simulink model "LoFT_Example3"  (R2024b)
settings: Solver=ode4  StartTime=0.0  StopTime=300  FixedStep=simu.dt  RelTol=1e-3
undefined symbols (not defined in the file): body, circtime, Communication, D1, Delta, irkb, line, LoFT, p0, Pn, s, simu, trip_time, Turbwind, waves, wind
libraries: simulink x350, spsThreePhaseVIMeasurementLib x41, spsThreePhasePISectionLineLib x34, spsThreePhaseParallelRLCLoadLib x21, spsThreePhaseTransformerTwoWindingsLib x14, spsLoadFlowBusLib x10, spsThreePhaseDynamicLoadLib x9, spsSynchronousMachinepuStandardLib x7, spsExcitationSystemLib x7, spsSteamTurbineandGovernorLib x7, spsGenericPowerSystemStabilizerLib x7, spsMultiBandPowerSystemStabilizerLib x7
(part 22 of 49)

== system LoFT_Example3/FOWT System/Subsystem5/FOWT5/Aerodynamics and Local Control Systems ==
  WindSpeed : Inport
  "Measureed " : Inport  Port=2
  Nacelle Speed : Inport  Port=3
  Power : Inport  Port=4
  Blade Pitch : Inport  Port=5
  Switch : Inport  Port=6
  Constant1 : Constant  Value=90*pi/180
  Demux : Demux  Outputs=2
  Divide3 : Product  Inputs=*/
  Hull Aerodynamic : Subsystem
  Local Control Systems : Subsystem
  Mux : Mux
  Mux1 : Mux
  Product : Product
  Rate Limiter : RateLimiter  RisingSlewLimit=Controller.torqueMaxRate  FallingSlewLimit=-Controller.torqueMaxRate  SampleTimeMode=inherited
  Rotor/drivetrain dynamics : Subsystem
  Saturation Dynamic : simulink/Discontinuities/Saturation Dynamic  OutMin=[]  OutMax=[]  OutDataTypeStr=Inherit: Same as second input  OutDataType=fixdt(1, 16)  OutScaling=2^-10  DoSatur=off
  Saturation2 : Saturate  UpperLimit=Controller.torqueMax  LowerLimit=0
  Switch1 : Switch  Criteria=u2 > Threshold  SaturateOnIntegerOverflow=off  InputSameDT=off
  Transfer Fcn : TransferFcn  Denominator=[0.2 1]
  smooth1 : Subsystem
  wind speed estimator : Subsystem
  Nacelle : Outport
  drivetrain : Outport  Port=2
  F_aero : Outport  Port=3
  wires:
  Transfer Fcn/1 -> [BldPitch]
  Mux1/1 -> drivetrain/1
  Mux/1 -> Nacelle/1
  Local Control Systems/2(BldPitch) -> Saturation Dynamic/2
  Saturation Dynamic/1 -> Transfer Fcn/1
  Switch/1 -> Demux/1
  [RotSpeed] -> Divide3/2
  Rate Limiter/1 -> Saturation2/1
  Switch1/1 -> Rate Limiter/1
  Local Control Systems/1(GenTorq) -> Switch1/3
  Divide3/1 -> Switch1/1
  Nacelle Speed/1 -> Local Control Systems/3(Nacelle Speed)
  [RotSpeed] -> Local Control Systems/2(RotSpeed)
  Power/1 -> smooth1/1(In1)
  Blade Pitch/1 -> Saturation Dynamic/3
  Saturation2/1 -> [GenTorq]
  smooth1/1(Out1) -> Divide3/1
  WindSpeed/1 -> [EffectiveWS]
  [EffectiveWS] -> Hull Aerodynamic/1(In1)
  [RotSpeed] -> Hull Aerodynamic/2(In2)
  [BldPitch] -> Hull Aerodynamic/3(In4)
  Hull Aerodynamic/1(Out1) -> F_aero/1
  [RotSpeed] -> Rotor/drivetrain dynamics/1(In1)
  [EffectiveWS] -> Rotor/drivetrain dynamics/2(In2)
  [BldPitch] -> Rotor/drivetrain dynamics/3(In3)
  [EffectiveWS] -> Rotor/drivetrain dynamics/4(In4)
  [GenTorq] -> Rotor/drivetrain dynamics/5(In5)
  Rotor/drivetrain dynamics/1(Out1) -> [RotSpeed]
  [EffectiveWS] -> Mux/1
  [MeasuredWS] -> Local Control Systems/1(WindSpeed)
  "Measureed "/1 -> [MeasuredWS]
  [MeasuredWS] -> wind speed estimator/1(In1)
  wind speed estimator/1(Out1) -> Mux/2
  [BldPitch] -> Mux/4
  Hull Aerodynamic/2(Rotor thrust) -> [RotorThrust]
  [RotorThrust] -> Mux/3
  Demux/1 -> Switch1/2
  [RotSpeed] -> Mux1/1, Product/1
  [GenTorq] -> Mux1/2, Product/2
  Product/1 -> Mux1/3
  Rotor/drivetrain dynamics/2(Out2) -> [RotTorq]
  [RotTorq] -> Mux1/4
  Constant1/1 -> Saturation Dynamic/1

== system LoFT_Example3/FOWT System/Subsystem5/FOWT5/Hydrodynamics ==
  Acceleration : Inport
  Speed : Inport  Port=2
  Position : Inport  Port=3
  Wave : Inport  Port=4
  Add : Sum  Inputs=--+
  excitation force : Subsystem
  radiation force : Subsystem
  "viscous force " : Subsystem
  Out1 : Outport
  wires:
  Wave/1 -> excitation force/2(Wave)
  Add/1 -> Out1/1
  excitation force/1(Fext) -> Add/3
  "viscous force "/1(F_vis) -> Add/2
  radiation force/1(F_rad) -> Add/1
  Position/1 -> excitation force/1(position)
  Acceleration/1 -> radiation force/1(velocity)
  Speed/1 -> "viscous force "/1(In1), radiation force/2(In2)

== system LoFT_Example3/FOWT System/Subsystem5/FOWT5/Hydrostatics ==
  position : Inport
  Add : Sum
  Add2 : Sum  Inputs=+--
  Assignment : Assignment  DiagnosticForDimensions=Warning  IndexOptions=Index vector (dialog)  Indices=2  OutputSizes=1
  Constant : Constant  Value=Property.masstot-9.7e6
  Constant1 : Constant  Value=Property.volume
  Constant2 : Constant  Value=[0 0 0]
  Constant3 : Constant  Value=4*445087
  Product : Product  Multiplication=Matrix(*)
  "Surge,heave,pitch, Hydro stiffness (3×3)" : Constant  Value=Hydro.hydrostatic
  rho * g : Gain  Gain=1025*9.81
  rho * g1 : Gain  Gain=9.81
  Out1 : Outport
  wires:
  Add2/1 -> Assignment/2
  Add/1 -> Out1/1
  Assignment/1 -> Add/1
  Constant2/1 -> Assignment/1
  rho * g/1 -> Add2/2
  rho * g1/1 -> Add2/1
  Constant/1 -> rho * g1/1
  Product/1 -> Add/2
  Constant1/1 -> rho * g/1
  position/1 -> Product/2
  "Surge,heave,pitch, Hydro stiffness (3×3)"/1 -> Product/1
  Constant3/1 -> Add2/3

== system LoFT_Example3/FOWT System/Subsystem5/FOWT5/Measurements ==
  Nacelle : Inport
  drivetrain : Inport  Port=2
  platform : Inport  Port=3
  Bus Creator : BusCreator  Inputs=17
  Demux : Demux  Outputs=9
  Demux1 : Demux
  Demux2 : Demux
  Out1 : Outport
  wires:
  drivetrain/1 -> Demux2/1
  Demux2/4 -> Bus Creator/8  "RotTorq"
  Demux2/3 -> Bus Creator/7  "GenPwr"
  Demux2/2 -> Bus Creator/6  "GenTorq"
  Demux2/1 -> Bus Creator/5  "RotSpeed"
  Demux/1 -> Bus Creator/9  "PtfmSurge"
  Demux/2 -> Bus Creator/10  "PtfmHeave"
  Demux/3 -> Bus Creator/11  "PtfmPitch"
  Demux/4 -> Bus Creator/12  "PtfmTVxi"
  Demux/5 -> Bus Creator/13  "PtfmTVzi"
  Demux/6 -> Bus Creator/14  "PtfmRVyi"
  Demux/7 -> Bus Creator/15  "PtfmTAxi"
  Demux/8 -> Bus Creator/16  "PtfmTAzi"
  Demux/9 -> Bus Creator/17  "PtfmRAyi"
  Demux1/1 -> Bus Creator/1  "WindVelX"
  Demux1/2 -> Bus Creator/2  "WindEst"
  Demux1/3 -> Bus Creator/3  "RotThrust"
  Demux1/4 -> Bus Creator/4  "BldPitch"
  Bus Creator/1 -> Out1/1
  Nacelle/1 -> Demux1/1
  platform/1 -> Demux/1

== system LoFT_Example3/FOWT System/Subsystem5/FOWT5/Moorings ==
  position : Inport
  2-D Lookup Table : Lookup_n-D  NumberOfTableDimensions=3  BreakpointsForDimension1=Mooring.X  BreakpointsForDimension2=Mooring.Z  BreakpointsForDimension3=Mooring.RY  Table=Mooring.FX  InternalRulePriority=Speed  RndMeth=Simplest
      settings: InputPortMap=u0,u1,u2
  2-D Lookup Table3 : Lookup_n-D  NumberOfTableDimensions=3  BreakpointsForDimension1=LoFT.Mooring.X  BreakpointsForDimension2=LoFT.Mooring.Z  BreakpointsForDimension3=LoFT.Mooring.RY  Table=LoFT.Mooring.FZ  InternalRulePriority=Speed  RndMeth=Simplest
      settings: InputPortMap=u0,u1,u2
  2-D Lookup Table4 : Lookup_n-D  NumberOfTableDimensions=3  BreakpointsForDimension1=LoFT.Mooring.X  BreakpointsForDimension2=LoFT.Mooring.Z  BreakpointsForDimension3=LoFT.Mooring.RY  Table=LoFT.Mooring.MY  InternalRulePriority=Speed  RndMeth=Simplest
      settings: InputPortMap=u0,u1,u2
  Demux : Demux  Outputs=3
  Demux1 : Demux  Outputs=3
  Demux2 : Demux  Outputs=3
  Vector Concatenate1 : Concatenate  NumInputs=3
  Out1 : Outport
  wires:
  Vector Concatenate1/1 -> Out1/1
  Demux2/2 -> 2-D Lookup Table4/2
  Demux2/1 -> 2-D Lookup Table4/1
  2-D Lookup Table4/1 -> Vector Concatenate1/3
  2-D Lookup Table3/1 -> Vector Concatenate1/2
  Demux1/3 -> 2-D Lookup Table3/3
  Demux/2 -> 2-D Lookup Table/2
  Demux1/1 -> 2-D Lookup Table3/1
  Demux2/3 -> 2-D Lookup Table4/3
  Demux/1 -> 2-D Lookup Table/1
  position/1 -> Demux/1, Demux1/1, Demux2/1
  2-D Lookup Table/1 -> Vector Concatenate1/1
  Demux1/2 -> 2-D Lookup Table3/2
  Demux/3 -> 2-D Lookup Table/3

== system LoFT_Example3/FOWT System/Subsystem5/FOWT5/Subsystem1 ==
  In1 : Inport
  In2 : Inport  Port=2
  In3 : Inport  Port=3
  In4 : Inport  Port=4
  In5 : Inport  Port=5
  In6 : Inport  Port=6
  Demux : Demux  Outputs=2
  Demux1 : Demux  Outputs=2
  Demux2 : Demux  Outputs=2
  Mux : Mux  Inputs=9
  Vector Concatenate : Concatenate
  Vector Concatenate1 : Concatenate
  Vector Concatenate2 : Concatenate
  Out4 : Outport
  Out1 : Outport  Port=2
  Out2 : Outport  Port=3
  Out3 : Outport  Port=4
  wires:
  Demux2/2 -> Mux/8
  Demux2/1 -> Mux/7
  Demux1/2 -> Mux/5
  Demux1/1 -> Mux/4
  Demux/2 -> Mux/2
  Demux/1 -> Mux/1
  Mux/1 -> Out4/1
  In6/1 -> Vector Concatenate2/1, Demux2/1
  In2/1 -> Vector Concatenate1/2, Mux/6
  In5/1 -> Vector Concatenate1/1, Demux1/1
  Vector Concatenate/1 -> Out1/1
  Vector Concatenate1/1 -> Out2/1
  Vector Concatenate2/1 -> Out3/1
  In4/1 -> Vector Concatenate/1, Demux/1
  In1/1 -> Vector Concatenate/2, Mux/3
  In3/1 -> Vector Concatenate2/2, Mux/9

== system LoFT_Example3/FOWT System/Subsystem5/FOWT5/wind speed(m//s) ==
  Inflow : Inport
  In2 : Inport  Port=2
  Add : Sum
  Demux : Demux  Outputs=3
  Product : Product
  Trigonometric Function : Trigonometry  Operator=cos
  add : Sum  Inputs=+-
  add1 : Sum  Inputs=+-
  hub height : Gain  Gain=145
  smooth1 : Subsystem  Commented=on
  Effective : Outport
  Measured : Outport  Port=2
  FB : Outport  Port=3
  wires:
  In2/1 -> Demux/1
  hub height/1 -> Product/1
  Trigonometric Function/1 -> Product/2
  Demux/1 -> Add/1
  Demux/3 -> hub height/1, Trigonometric Function/1
  add/1 -> Effective/1
  add1/1 -> Measured/1
  Product/1 -> Add/2
  Add/1 -> [HubVelocity]
  [HubVelocity] -> add1/2
  [HubVelocity] -> add/2
  [HubVelocity] -> FB/1
  Inflow/1 -> add1/1, add/1

== system LoFT_Example3/FOWT System/Subsystem5/FOWT6/Aerodynamics and Local Control Systems ==
  WindSpeed : Inport
  "Measureed " : Inport  Port=2
  Nacelle Speed : Inport  Port=3
  Power : Inport  Port=4
  Blade Pitch : Inport  Port=5
  Switch : Inport  Port=6
  Constant1 : Constant  Value=90*pi/180
  Demux : Demux  Outputs=2
  Divide3 : Product  Inputs=*/
  Hull Aerodynamic : Subsystem
  Local Control Systems : Subsystem
  Mux : Mux
  Mux1 : Mux
  Product : Product
  Rate Limiter : RateLimiter  RisingSlewLimit=Controller.torqueMaxRate  FallingSlewLimit=-Controller.torqueMaxRate  SampleTimeMode=inherited
  Rotor/drivetrain dynamics : Subsystem
  Saturation Dynamic : simulink/Discontinuities/Saturation Dynamic  OutMin=[]  OutMax=[]  OutDataTypeStr=Inherit: Same as second input  OutDataType=fixdt(1, 16)  OutScaling=2^-10  DoSatur=off
  Saturation2 : Saturate  UpperLimit=Controller.torqueMax  LowerLimit=0
  Switch1 : Switch  Criteria=u2 > Threshold  SaturateOnIntegerOverflow=off  InputSameDT=off
  Transfer Fcn : TransferFcn  Denominator=[0.2 1]
  smooth1 : Subsystem
  wind speed estimator : Subsystem
  Nacelle : Outport
  drivetrain : Outport  Port=2
  F_aero : Outport  Port=3
  wires:
  Constant1/1 -> Saturation Dynamic/1
  [RotTorq] -> Mux1/4
  Rotor/drivetrain dynamics/2(Out2) -> [RotTorq]
  Product/1 -> Mux1/3
  [GenTorq] -> Product/2, Mux1/2
  [RotSpeed] -> Product/1, Mux1/1
  Demux/1 -> Switch1/2
  [RotorThrust] -> Mux/3
  Hull Aerodynamic/2(Rotor thrust) -> [RotorThrust]
  [BldPitch] -> Mux/4
  wind speed estimator/1(Out1) -> Mux/2
  [MeasuredWS] -> wind speed estimator/1(In1)
  "Measureed "/1 -> [MeasuredWS]
  [MeasuredWS] -> Local Control Systems/1(WindSpeed)
  [EffectiveWS] -> Mux/1
  Rotor/drivetrain dynamics/1(Out1) -> [RotSpeed]
  [GenTorq] -> Rotor/drivetrain dynamics/5(In5)
  [EffectiveWS] -> Rotor/drivetrain dynamics/4(In4)
  [BldPitch] -> Rotor/drivetrain dynamics/3(In3)
  [EffectiveWS] -> Rotor/drivetrain dynamics/2(In2)
  [RotSpeed] -> Rotor/drivetrain dynamics/1(In1)
  Hull Aerodynamic/1(Out1) -> F_aero/1
  [BldPitch] -> Hull Aerodynamic/3(In4)
  [RotSpeed] -> Hull Aerodynamic/2(In2)
  [EffectiveWS] -> Hull Aerodynamic/1(In1)
  WindSpeed/1 -> [EffectiveWS]
  smooth1/1(Out1) -> Divide3/1
  Saturation2/1 -> [GenTorq]
  Blade Pitch/1 -> Saturation Dynamic/3
  Power/1 -> smooth1/1(In1)
  [RotSpeed] -> Local Control Systems/2(RotSpeed)
  Nacelle Speed/1 -> Local Control Systems/3(Nacelle Speed)
  Divide3/1 -> Switch1/1
  Local Control Systems/1(GenTorq) -> Switch1/3
  Switch1/1 -> Rate Limiter/1
  Rate Limiter/1 -> Saturation2/1
  [RotSpeed] -> Divide3/2
  Switch/1 -> Demux/1
  Saturation Dynamic/1 -> Transfer Fcn/1
  Local Control Systems/2(BldPitch) -> Saturation Dynamic/2
  Mux/1 -> Nacelle/1
  Mux1/1 -> drivetrain/1
  Transfer Fcn/1 -> [BldPitch]

== system LoFT_Example3/FOWT System/Subsystem5/FOWT6/Hydrodynamics ==
  Acceleration : Inport
  Speed : Inport  Port=2
  Position : Inport  Port=3
  Wave : Inport  Port=4
  Add : Sum  Inputs=--+
  excitation force : Subsystem
  radiation force : Subsystem
  "viscous force " : Subsystem
  Out1 : Outport
  wires:
  Speed/1 -> radiation force/2(In2), "viscous force "/1(In1)
  Acceleration/1 -> radiation force/1(velocity)
  Position/1 -> excitation force/1(position)
  radiation force/1(F_rad) -> Add/1
  "viscous force "/1(F_vis) -> Add/2
  excitation force/1(Fext) -> Add/3
  Add/1 -> Out1/1
  Wave/1 -> excitation force/2(Wave)

== system LoFT_Example3/FOWT System/Subsystem5/FOWT6/Hydrostatics ==
  position : Inport
  Add : Sum
  Add2 : Sum  Inputs=+--
  Assignment : Assignment  DiagnosticForDimensions=Warning  IndexOptions=Index vector (dialog)  Indices=2  OutputSizes=1
  Constant : Constant  Value=Property.masstot-9.7e6
  Constant1 : Constant  Value=Property.volume
  Constant2 : Constant  Value=[0 0 0]
  Constant3 : Constant  Value=4*445087
  Product : Product  Multiplication=Matrix(*)
  "Surge,heave,pitch, Hydro stiffness (3×3)" : Constant  Value=Hydro.hydrostatic
  rho * g : Gain  Gain=1025*9.81
  rho * g1 : Gain  Gain=9.81
  Out1 : Outport
  wires:
  Constant3/1 -> Add2/3
  "Surge,heave,pitch, Hydro stiffness (3×3)"/1 -> Product/1
  position/1 -> Product/2
  Constant1/1 -> rho * g/1
  Product/1 -> Add/2
  Constant/1 -> rho * g1/1
  rho * g1/1 -> Add2/1
  rho * g/1 -> Add2/2
  Constant2/1 -> Assignment/1
  Assignment/1 -> Add/1
  Add/1 -> Out1/1
  Add2/1 -> Assignment/2

== system LoFT_Example3/FOWT System/Subsystem5/FOWT6/Measurements ==
  Nacelle : Inport
  drivetrain : Inport  Port=2
  platform : Inport  Port=3
  Bus Creator : BusCreator  Inputs=17
  Demux : Demux  Outputs=9
  Demux1 : Demux
  Demux2 : Demux
  Out1 : Outport
  wires:
  platform/1 -> Demux/1
  Nacelle/1 -> Demux1/1
  Bus Creator/1 -> Out1/1
  Demux1/4 -> Bus Creator/4  "BldPitch"
  Demux1/3 -> Bus Creator/3  "RotThrust"
  Demux1/2 -> Bus Creator/2  "WindEst"
  Demux1/1 -> Bus Creator/1  "WindVelX"
  Demux/9 -> Bus Creator/17  "PtfmRAyi"
  Demux/8 -> Bus Creator/16  "PtfmTAzi"
  Demux/7 -> Bus Creator/15  "PtfmTAxi"
  Demux/6 -> Bus Creator/14  "PtfmRVyi"
  Demux/5 -> Bus Creator/13  "PtfmTVzi"
  Demux/4 -> Bus Creator/12  "PtfmTVxi"
  Demux/3 -> Bus Creator/11  "PtfmPitch"
  Demux/2 -> Bus Creator/10  "PtfmHeave"
  Demux/1 -> Bus Creator/9  "PtfmSurge"
  Demux2/1 -> Bus Creator/5  "RotSpeed"
  Demux2/2 -> Bus Creator/6  "GenTorq"
  Demux2/3 -> Bus Creator/7  "GenPwr"
  Demux2/4 -> Bus Creator/8  "RotTorq"
  drivetrain/1 -> Demux2/1

== system LoFT_Example3/FOWT System/Subsystem5/FOWT6/Moorings ==
  position : Inport
  2-D Lookup Table : Lookup_n-D  NumberOfTableDimensions=3  BreakpointsForDimension1=Mooring.X  BreakpointsForDimension2=Mooring.Z  BreakpointsForDimension3=Mooring.RY  Table=Mooring.FX  InternalRulePriority=Speed  RndMeth=Simplest
      settings: InputPortMap=u0,u1,u2
  2-D Lookup Table3 : Lookup_n-D  NumberOfTableDimensions=3  BreakpointsForDimension1=LoFT.Mooring.X  BreakpointsForDimension2=LoFT.Mooring.Z  BreakpointsForDimension3=LoFT.Mooring.RY  Table=LoFT.Mooring.FZ  InternalRulePriority=Speed  RndMeth=Simplest
      settings: InputPortMap=u0,u1,u2
  2-D Lookup Table4 : Lookup_n-D  NumberOfTableDimensions=3  BreakpointsForDimension1=LoFT.Mooring.X  BreakpointsForDimension2=LoFT.Mooring.Z  BreakpointsForDimension3=LoFT.Mooring.RY  Table=LoFT.Mooring.MY  InternalRulePriority=Speed  RndMeth=Simplest
      settings: InputPortMap=u0,u1,u2
  Demux : Demux  Outputs=3
  Demux1 : Demux  Outputs=3
  Demux2 : Demux  Outputs=3
  Vector Concatenate1 : Concatenate  NumInputs=3
  Out1 : Outport
  wires:
  Demux/3 -> 2-D Lookup Table/3
  Demux1/2 -> 2-D Lookup Table3/2
  2-D Lookup Table/1 -> Vector Concatenate1/1
  position/1 -> Demux2/1, Demux1/1, Demux/1
  Demux/1 -> 2-D Lookup Table/1
  Demux2/3 -> 2-D Lookup Table4/3
  Demux1/1 -> 2-D Lookup Table3/1
  Demux/2 -> 2-D Lookup Table/2
  Demux1/3 -> 2-D Lookup Table3/3
  2-D Lookup Table3/1 -> Vector Concatenate1/2
  2-D Lookup Table4/1 -> Vector Concatenate1/3
  Demux2/1 -> 2-D Lookup Table4/1
  Demux2/2 -> 2-D Lookup Table4/2
  Vector Concatenate1/1 -> Out1/1

== system LoFT_Example3/FOWT System/Subsystem5/FOWT6/Subsystem1 ==
  In1 : Inport
  In2 : Inport  Port=2
  In3 : Inport  Port=3
  In4 : Inport  Port=4
  In5 : Inport  Port=5
  In6 : Inport  Port=6
  Demux : Demux  Outputs=2
  Demux1 : Demux  Outputs=2
  Demux2 : Demux  Outputs=2
  Mux : Mux  Inputs=9
  Vector Concatenate : Concatenate
  Vector Concatenate1 : Concatenate
  Vector Concatenate2 : Concatenate
  Out4 : Outport
  Out1 : Outport  Port=2
  Out2 : Outport  Port=3
  Out3 : Outport  Port=4
  wires:
  In3/1 -> Mux/9, Vector Concatenate2/2
  In1/1 -> Mux/3, Vector Concatenate/2
  In4/1 -> Demux/1, Vector Concatenate/1
  Vector Concatenate2/1 -> Out3/1
  Vector Concatenate1/1 -> Out2/1
  Vector Concatenate/1 -> Out1/1
  In5/1 -> Demux1/1, Vector Concatenate1/1
  In2/1 -> Mux/6, Vector Concatenate1/2
  In6/1 -> Demux2/1, Vector Concatenate2/1
  Mux/1 -> Out4/1
  Demux/1 -> Mux/1
  Demux/2 -> Mux/2
  Demux1/1 -> Mux/4
  Demux1/2 -> Mux/5
  Demux2/1 -> Mux/7
  Demux2/2 -> Mux/8

== system LoFT_Example3/FOWT System/Subsystem5/FOWT6/wind speed(m//s) ==
  Inflow : Inport
  In2 : Inport  Port=2
  Add : Sum
  Demux : Demux  Outputs=3
  Product : Product
  Trigonometric Function : Trigonometry  Operator=cos
  add : Sum  Inputs=+-
  add1 : Sum  Inputs=+-
  hub height : Gain  Gain=145
  smooth1 : Subsystem  Commented=on
  Effective : Outport
  Measured : Outport  Port=2
  FB : Outport  Port=3
  wires:
  Inflow/1 -> add/1, add1/1
  [HubVelocity] -> FB/1
  [HubVelocity] -> add/2
  [HubVelocity] -> add1/2
  Add/1 -> [HubVelocity]
  Product/1 -> Add/2
  add1/1 -> Measured/1
  add/1 -> Effective/1
  Demux/3 -> Trigonometric Function/1, hub height/1
  Demux/1 -> Add/1
  Trigonometric Function/1 -> Product/2
  hub height/1 -> Product/1
  In2/1 -> Demux/1

== system LoFT_Example3/FOWT System/Subsystem5/FOWT7/Aerodynamics and Local Control Systems ==
  WindSpeed : Inport
  "Measureed " : Inport  Port=2
  Nacelle Speed : Inport  Port=3
  Power : Inport  Port=4
  Blade Pitch : Inport  Port=5
  Switch : Inport  Port=6
  Constant1 : Constant  Value=90*pi/180
  Demux : Demux  Outputs=2
  Divide3 : Product  Inputs=*/
  Hull Aerodynamic : Subsystem
  Local Control Systems : Subsystem
  Mux : Mux
  Mux1 : Mux
  Product : Product
  Rate Limiter : RateLimiter  RisingSlewLimit=Controller.torqueMaxRate  FallingSlewLimit=-Controller.torqueMaxRate  SampleTimeMode=inherited
  Rotor/drivetrain dynamics : Subsystem
  Saturation Dynamic : simulink/Discontinuities/Saturation Dynamic  OutMin=[]  OutMax=[]  OutDataTypeStr=Inherit: Same as second input  OutDataType=fixdt(1, 16)  OutScaling=2^-10  DoSatur=off
  Saturation2 : Saturate  UpperLimit=Controller.torqueMax  LowerLimit=0
  Switch1 : Switch  Criteria=u2 > Threshold  SaturateOnIntegerOverflow=off  InputSameDT=off
  Transfer Fcn : TransferFcn  Denominator=[0.2 1]
  smooth1 : Subsystem
  wind speed estimator : Subsystem
  Nacelle : Outport
  drivetrain : Outport  Port=2
  F_aero : Outport  Port=3
  wires:
  Transfer Fcn/1 -> [BldPitch]
  Mux1/1 -> drivetrain/1
  Mux/1 -> Nacelle/1
  Local Control Systems/2(BldPitch) -> Saturation Dynamic/2
  Saturation Dynamic/1 -> Transfer Fcn/1
  Switch/1 -> Demux/1
  [RotSpeed] -> Divide3/2
  Rate Limiter/1 -> Saturation2/1
  Switch1/1 -> Rate Limiter/1
  Local Control Systems/1(GenTorq) -> Switch1/3
  Divide3/1 -> Switch1/1
  Nacelle Speed/1 -> Local Control Systems/3(Nacelle Speed)
  [RotSpeed] -> Local Control Systems/2(RotSpeed)
  Power/1 -> smooth1/1(In1)
  Blade Pitch/1 -> Saturation Dynamic/3
  Saturation2/1 -> [GenTorq]
  smooth1/1(Out1) -> Divide3/1
  WindSpeed/1 -> [EffectiveWS]
  [EffectiveWS] -> Hull Aerodynamic/1(In1)
  [RotSpeed] -> Hull Aerodynamic/2(In2)
  [BldPitch] -> Hull Aerodynamic/3(In4)
  Hull Aerodynamic/1(Out1) -> F_aero/1
  [RotSpeed] -> Rotor/drivetrain dynamics/1(In1)
  [EffectiveWS] -> Rotor/drivetrain dynamics/2(In2)
  [BldPitch] -> Rotor/drivetrain dynamics/3(In3)
  [EffectiveWS] -> Rotor/drivetrain dynamics/4(In4)
  [GenTorq] -> Rotor/drivetrain dynamics/5(In5)
  Rotor/drivetrain dynamics/1(Out1) -> [RotSpeed]
  [EffectiveWS] -> Mux/1
  [MeasuredWS] -> Local Control Systems/1(WindSpeed)
  "Measureed "/1 -> [MeasuredWS]
  [MeasuredWS] -> wind speed estimator/1(In1)
  wind speed estimator/1(Out1) -> Mux/2
  [BldPitch] -> Mux/4
  Hull Aerodynamic/2(Rotor thrust) -> [RotorThrust]
  [RotorThrust] -> Mux/3
  Demux/1 -> Switch1/2
  [RotSpeed] -> Mux1/1, Product/1
  [GenTorq] -> Mux1/2, Product/2
  Product/1 -> Mux1/3
  Rotor/drivetrain dynamics/2(Out2) -> [RotTorq]
  [RotTorq] -> Mux1/4
  Constant1/1 -> Saturation Dynamic/1

== system LoFT_Example3/FOWT System/Subsystem5/FOWT7/Hydrodynamics ==
  Acceleration : Inport
  Speed : Inport  Port=2
  Position : Inport  Port=3
  Wave : Inport  Port=4
  Add : Sum  Inputs=--+
  excitation force : Subsystem
  radiation force : Subsystem
  "viscous force " : Subsystem
  Out1 : Outport
  wires:
  Wave/1 -> excitation force/2(Wave)
  Add/1 -> Out1/1
  excitation force/1(Fext) -> Add/3
  "viscous force "/1(F_vis) -> Add/2
  radiation force/1(F_rad) -> Add/1
  Position/1 -> excitation force/1(position)
  Acceleration/1 -> radiation force/1(velocity)
  Speed/1 -> "viscous force "/1(In1), radiation force/2(In2)

== system LoFT_Example3/FOWT System/Subsystem5/FOWT7/Hydrostatics ==
  position : Inport
  Add : Sum
  Add2 : Sum  Inputs=+--
  Assignment : Assignment  DiagnosticForDimensions=Warning  IndexOptions=Index vector (dialog)  Indices=2  OutputSizes=1
  Constant : Constant  Value=Property.masstot-9.7e6
  Constant1 : Constant  Value=Property.volume
  Constant2 : Constant  Value=[0 0 0]
  Constant3 : Constant  Value=4*445087
  Product : Product  Multiplication=Matrix(*)
  "Surge,heave,pitch, Hydro stiffness (3×3)" : Constant  Value=Hydro.hydrostatic
  rho * g : Gain  Gain=1025*9.81
  rho * g1 : Gain  Gain=9.81
  Out1 : Outport
  wires:
  Add2/1 -> Assignment/2
  Add/1 -> Out1/1
  Assignment/1 -> Add/1
  Constant2/1 -> Assignment/1
  rho * g/1 -> Add2/2
  rho * g1/1 -> Add2/1
  Constant/1 -> rho * g1/1
  Product/1 -> Add/2
  Constant1/1 -> rho * g/1
  position/1 -> Product/2
  "Surge,heave,pitch, Hydro stiffness (3×3)"/1 -> Product/1
  Constant3/1 -> Add2/3

== system LoFT_Example3/FOWT System/Subsystem5/FOWT7/Measurements ==
  Nacelle : Inport
  drivetrain : Inport  Port=2
  platform : Inport  Port=3
  Bus Creator : BusCreator  Inputs=17
  Demux : Demux  Outputs=9
  Demux1 : Demux
  Demux2 : Demux
  Out1 : Outport
  wires:
  drivetrain/1 -> Demux2/1
  Demux2/4 -> Bus Creator/8  "RotTorq"
  Demux2/3 -> Bus Creator/7  "GenPwr"
  Demux2/2 -> Bus Creator/6  "GenTorq"
  Demux2/1 -> Bus Creator/5  "RotSpeed"
  Demux/1 -> Bus Creator/9  "PtfmSurge"
  Demux/2 -> Bus Creator/10  "PtfmHeave"
  Demux/3 -> Bus Creator/11  "PtfmPitch"
  Demux/4 -> Bus Creator/12  "PtfmTVxi"
  Demux/5 -> Bus Creator/13  "PtfmTVzi"
  Demux/6 -> Bus Creator/14  "PtfmRVyi"
  Demux/7 -> Bus Creator/15  "PtfmTAxi"
  Demux/8 -> Bus Creator/16  "PtfmTAzi"
  Demux/9 -> Bus Creator/17  "PtfmRAyi"
  Demux1/1 -> Bus Creator/1  "WindVelX"
  Demux1/2 -> Bus Creator/2  "WindEst"
  Demux1/3 -> Bus Creator/3  "RotThrust"
  Demux1/4 -> Bus Creator/4  "BldPitch"
  Bus Creator/1 -> Out1/1
  Nacelle/1 -> Demux1/1
  platform/1 -> Demux/1

== system LoFT_Example3/FOWT System/Subsystem5/FOWT7/Moorings ==
  position : Inport
  2-D Lookup Table : Lookup_n-D  NumberOfTableDimensions=3  BreakpointsForDimension1=Mooring.X  BreakpointsForDimension2=Mooring.Z  BreakpointsForDimension3=Mooring.RY  Table=Mooring.FX  InternalRulePriority=Speed  RndMeth=Simplest
      settings: InputPortMap=u0,u1,u2
  2-D Lookup Table3 : Lookup_n-D  NumberOfTableDimensions=3  BreakpointsForDimension1=LoFT.Mooring.X  BreakpointsForDimension2=LoFT.Mooring.Z  BreakpointsForDimension3=LoFT.Mooring.RY  Table=LoFT.Mooring.FZ  InternalRulePriority=Speed  RndMeth=Simplest
      settings: InputPortMap=u0,u1,u2
  2-D Lookup Table4 : Lookup_n-D  NumberOfTableDimensions=3  BreakpointsForDimension1=LoFT.Mooring.X  BreakpointsForDimension2=LoFT.Mooring.Z  BreakpointsForDimension3=LoFT.Mooring.RY  Table=LoFT.Mooring.MY  InternalRulePriority=Speed  RndMeth=Simplest
      settings: InputPortMap=u0,u1,u2
  Demux : Demux  Outputs=3
  Demux1 : Demux  Outputs=3
  Demux2 : Demux  Outputs=3
  Vector Concatenate1 : Concatenate  NumInputs=3
  Out1 : Outport
  wires:
  Vector Concatenate1/1 -> Out1/1
  Demux2/2 -> 2-D Lookup Table4/2
  Demux2/1 -> 2-D Lookup Table4/1
  2-D Lookup Table4/1 -> Vector Concatenate1/3
  2-D Lookup Table3/1 -> Vector Concatenate1/2
  Demux1/3 -> 2-D Lookup Table3/3
  Demux/2 -> 2-D Lookup Table/2
  Demux1/1 -> 2-D Lookup Table3/1
  Demux2/3 -> 2-D Lookup Table4/3
  Demux/1 -> 2-D Lookup Table/1
  position/1 -> Demux/1, Demux1/1, Demux2/1
  2-D Lookup Table/1 -> Vector Concatenate1/1
  Demux1/2 -> 2-D Lookup Table3/2
  Demux/3 -> 2-D Lookup Table/3

== system LoFT_Example3/FOWT System/Subsystem5/FOWT7/Subsystem1 ==
  In1 : Inport
  In2 : Inport  Port=2
  In3 : Inport  Port=3
  In4 : Inport  Port=4
  In5 : Inport  Port=5
  In6 : Inport  Port=6
  Demux : Demux  Outputs=2
  Demux1 : Demux  Outputs=2
  Demux2 : Demux  Outputs=2
  Mux : Mux  Inputs=9
  Vector Concatenate : Concatenate
  Vector Concatenate1 : Concatenate
  Vector Concatenate2 : Concatenate
  Out4 : Outport
  Out1 : Outport  Port=2
  Out2 : Outport  Port=3
  Out3 : Outport  Port=4
  wires:
  Demux2/2 -> Mux/8
  Demux2/1 -> Mux/7
  Demux1/2 -> Mux/5
  Demux1/1 -> Mux/4
  Demux/2 -> Mux/2
  Demux/1 -> Mux/1
  Mux/1 -> Out4/1
  In6/1 -> Vector Concatenate2/1, Demux2/1
  In2/1 -> Vector Concatenate1/2, Mux/6
  In5/1 -> Vector Concatenate1/1, Demux1/1
  Vector Concatenate/1 -> Out1/1
  Vector Concatenate1/1 -> Out2/1
  Vector Concatenate2/1 -> Out3/1
  In4/1 -> Vector Concatenate/1, Demux/1
  In1/1 -> Vector Concatenate/2, Mux/3
  In3/1 -> Vector Concatenate2/2, Mux/9

== system LoFT_Example3/FOWT System/Subsystem5/FOWT7/wind speed(m//s) ==
  Inflow : Inport
  In2 : Inport  Port=2
  Add : Sum
  Demux : Demux  Outputs=3
  Product : Product
  Trigonometric Function : Trigonometry  Operator=cos
  add : Sum  Inputs=+-
  add1 : Sum  Inputs=+-
  hub height : Gain  Gain=145
  smooth1 : Subsystem  Commented=on
  Effective : Outport
  Measured : Outport  Port=2
  FB : Outport  Port=3
  wires:
  In2/1 -> Demux/1
  hub height/1 -> Product/1
  Trigonometric Function/1 -> Product/2
  Demux/1 -> Add/1
  Demux/3 -> hub height/1, Trigonometric Function/1
  add/1 -> Effective/1
  add1/1 -> Measured/1
  Product/1 -> Add/2
  Add/1 -> [HubVelocity]
  [HubVelocity] -> add1/2
  [HubVelocity] -> add/2
  [HubVelocity] -> FB/1
  Inflow/1 -> add1/1, add/1

== system LoFT_Example3/FOWT System/Subsystem5/FOWT8/Aerodynamics and Local Control Systems ==
  WindSpeed : Inport
  "Measureed " : Inport  Port=2
  Nacelle Speed : Inport  Port=3
  Power : Inport  Port=4
  Blade Pitch : Inport  Port=5
  Switch : Inport  Port=6
  Constant1 : Constant  Value=90*pi/180
  Demux : Demux  Outputs=2
  Divide3 : Product  Inputs=*/
  Hull Aerodynamic : Subsystem
  Local Control Systems : Subsystem
  Mux : Mux
  Mux1 : Mux
  Product : Product
  Rate Limiter : RateLimiter  RisingSlewLimit=Controller.torqueMaxRate  FallingSlewLimit=-Controller.torqueMaxRate  SampleTimeMode=inherited
  Rotor/drivetrain dynamics : Subsystem
  Saturation Dynamic : simulink/Discontinuities/Saturation Dynamic  OutMin=[]  OutMax=[]  OutDataTypeStr=Inherit: Same as second input  OutDataType=fixdt(1, 16)  OutScaling=2^-10  DoSatur=off
  Saturation2 : Saturate  UpperLimit=Controller.torqueMax  LowerLimit=0
  Switch1 : Switch  Criteria=u2 > Threshold  SaturateOnIntegerOverflow=off  InputSameDT=off
  Transfer Fcn : TransferFcn  Denominator=[0.2 1]
  smooth1 : Subsystem
  wind speed estimator : Subsystem
  Nacelle : Outport
  drivetrain : Outport  Port=2
  F_aero : Outport  Port=3
  wires:
  Constant1/1 -> Saturation Dynamic/1
  [RotTorq] -> Mux1/4
  Rotor/drivetrain dynamics/2(Out2) -> [RotTorq]
  Product/1 -> Mux1/3
  [GenTorq] -> Product/2, Mux1/2
  [RotSpeed] -> Product/1, Mux1/1
  Demux/1 -> Switch1/2
  [RotorThrust] -> Mux/3
  Hull Aerodynamic/2(Rotor thrust) -> [RotorThrust]
  [BldPitch] -> Mux/4
  wind speed estimator/1(Out1) -> Mux/2
  [MeasuredWS] -> wind speed estimator/1(In1)
  "Measureed "/1 -> [MeasuredWS]
  [MeasuredWS] -> Local Control Systems/1(WindSpeed)
  [EffectiveWS] -> Mux/1
  Rotor/drivetrain dynamics/1(Out1) -> [RotSpeed]
  [GenTorq] -> Rotor/drivetrain dynamics/5(In5)
  [EffectiveWS] -> Rotor/drivetrain dynamics/4(In4)
  [BldPitch] -> Rotor/drivetrain dynamics/3(In3)
  [EffectiveWS] -> Rotor/drivetrain dynamics/2(In2)
  [RotSpeed] -> Rotor/drivetrain dynamics/1(In1)
  Hull Aerodynamic/1(Out1) -> F_aero/1
  [BldPitch] -> Hull Aerodynamic/3(In4)
  [RotSpeed] -> Hull Aerodynamic/2(In2)
  [EffectiveWS] -> Hull Aerodynamic/1(In1)
  WindSpeed/1 -> [EffectiveWS]
  smooth1/1(Out1) -> Divide3/1
  Saturation2/1 -> [GenTorq]
  Blade Pitch/1 -> Saturation Dynamic/3
  Power/1 -> smooth1/1(In1)
  [RotSpeed] -> Local Control Systems/2(RotSpeed)
  Nacelle Speed/1 -> Local Control Systems/3(Nacelle Speed)
  Divide3/1 -> Switch1/1
  Local Control Systems/1(GenTorq) -> Switch1/3
  Switch1/1 -> Rate Limiter/1
  Rate Limiter/1 -> Saturation2/1
  [RotSpeed] -> Divide3/2
  Switch/1 -> Demux/1
  Saturation Dynamic/1 -> Transfer Fcn/1
  Local Control Systems/2(BldPitch) -> Saturation Dynamic/2
  Mux/1 -> Nacelle/1
  Mux1/1 -> drivetrain/1
  Transfer Fcn/1 -> [BldPitch]

== system LoFT_Example3/FOWT System/Subsystem5/FOWT8/Hydrodynamics ==
  Acceleration : Inport
  Speed : Inport  Port=2
  Position : Inport  Port=3
  Wave : Inport  Port=4
  Add : Sum  Inputs=--+
  excitation force : Subsystem
  radiation force : Subsystem
  "viscous force " : Subsystem
  Out1 : Outport
  wires:
  Speed/1 -> radiation force/2(In2), "viscous force "/1(In1)
  Acceleration/1 -> radiation force/1(velocity)
  Position/1 -> excitation force/1(position)
  radiation force/1(F_rad) -> Add/1
  "viscous force "/1(F_vis) -> Add/2
  excitation force/1(Fext) -> Add/3
  Add/1 -> Out1/1
  Wave/1 -> excitation force/2(Wave)

== system LoFT_Example3/FOWT System/Subsystem5/FOWT8/Hydrostatics ==
  position : Inport
  Add : Sum
  Add2 : Sum  Inputs=+--
  Assignment : Assignment  DiagnosticForDimensions=Warning  IndexOptions=Index vector (dialog)  Indices=2  OutputSizes=1
  Constant : Constant  Value=Property.masstot-9.7e6
  Constant1 : Constant  Value=Property.volume
  Constant2 : Constant  Value=[0 0 0]
  Constant3 : Constant  Value=4*445087
  Product : Product  Multiplication=Matrix(*)
  "Surge,heave,pitch, Hydro stiffness (3×3)" : Constant  Value=Hydro.hydrostatic
  rho * g : Gain  Gain=1025*9.81
  rho * g1 : Gain  Gain=9.81
  Out1 : Outport
  wires:
  Constant3/1 -> Add2/3
  "Surge,heave,pitch, Hydro stiffness (3×3)"/1 -> Product/1
  position/1 -> Product/2
  Constant1/1 -> rho * g/1
  Product/1 -> Add/2
  Constant/1 -> rho * g1/1
  rho * g1/1 -> Add2/1
  rho * g/1 -> Add2/2
  Constant2/1 -> Assignment/1
  Assignment/1 -> Add/1
  Add/1 -> Out1/1
  Add2/1 -> Assignment/2

== system LoFT_Example3/FOWT System/Subsystem5/FOWT8/Measurements ==
  Nacelle : Inport
  drivetrain : Inport  Port=2
  platform : Inport  Port=3
  Bus Creator : BusCreator  Inputs=17
  Demux : Demux  Outputs=9
  Demux1 : Demux
  Demux2 : Demux
  Out1 : Outport
  wires:
  platform/1 -> Demux/1
  Nacelle/1 -> Demux1/1
  Bus Creator/1 -> Out1/1
  Demux1/4 -> Bus Creator/4  "BldPitch"
  Demux1/3 -> Bus Creator/3  "RotThrust"
  Demux1/2 -> Bus Creator/2  "WindEst"
  Demux1/1 -> Bus Creator/1  "WindVelX"
  Demux/9 -> Bus Creator/17  "PtfmRAyi"
  Demux/8 -> Bus Creator/16  "PtfmTAzi"
  Demux/7 -> Bus Creator/15  "PtfmTAxi"
  Demux/6 -> Bus Creator/14  "PtfmRVyi"
  Demux/5 -> Bus Creator/13  "PtfmTVzi"
  Demux/4 -> Bus Creator/12  "PtfmTVxi"
  Demux/3 -> Bus Creator/11  "PtfmPitch"
  Demux/2 -> Bus Creator/10  "PtfmHeave"
  Demux/1 -> Bus Creator/9  "PtfmSurge"
  Demux2/1 -> Bus Creator/5  "RotSpeed"
  Demux2/2 -> Bus Creator/6  "GenTorq"
  Demux2/3 -> Bus Creator/7  "GenPwr"
  Demux2/4 -> Bus Creator/8  "RotTorq"
  drivetrain/1 -> Demux2/1

== system LoFT_Example3/FOWT System/Subsystem5/FOWT8/Moorings ==
  position : Inport
  2-D Lookup Table : Lookup_n-D  NumberOfTableDimensions=3  BreakpointsForDimension1=Mooring.X  BreakpointsForDimension2=Mooring.Z  BreakpointsForDimension3=Mooring.RY  Table=Mooring.FX  InternalRulePriority=Speed  RndMeth=Simplest
      settings: InputPortMap=u0,u1,u2
  2-D Lookup Table3 : Lookup_n-D  NumberOfTableDimensions=3  BreakpointsForDimension1=LoFT.Mooring.X  BreakpointsForDimension2=LoFT.Mooring.Z  BreakpointsForDimension3=LoFT.Mooring.RY  Table=LoFT.Mooring.FZ  InternalRulePriority=Speed  RndMeth=Simplest
      settings: InputPortMap=u0,u1,u2
  2-D Lookup Table4 : Lookup_n-D  NumberOfTableDimensions=3  BreakpointsForDimension1=LoFT.Mooring.X  BreakpointsForDimension2=LoFT.Mooring.Z  BreakpointsForDimension3=LoFT.Mooring.RY  Table=LoFT.Mooring.MY  InternalRulePriority=Speed  RndMeth=Simplest
      settings: InputPortMap=u0,u1,u2
  Demux : Demux  Outputs=3
  Demux1 : Demux  Outputs=3
  Demux2 : Demux  Outputs=3
  Vector Concatenate1 : Concatenate  NumInputs=3
  Out1 : Outport
  wires:
  Demux/3 -> 2-D Lookup Table/3
  Demux1/2 -> 2-D Lookup Table3/2
  2-D Lookup Table/1 -> Vector Concatenate1/1
  position/1 -> Demux2/1, Demux1/1, Demux/1
  Demux/1 -> 2-D Lookup Table/1
  Demux2/3 -> 2-D Lookup Table4/3
  Demux1/1 -> 2-D Lookup Table3/1
  Demux/2 -> 2-D Lookup Table/2
  Demux1/3 -> 2-D Lookup Table3/3
  2-D Lookup Table3/1 -> Vector Concatenate1/2
  2-D Lookup Table4/1 -> Vector Concatenate1/3
  Demux2/1 -> 2-D Lookup Table4/1
  Demux2/2 -> 2-D Lookup Table4/2
  Vector Concatenate1/1 -> Out1/1

== system LoFT_Example3/FOWT System/Subsystem5/FOWT8/Subsystem1 ==
  In1 : Inport
  In2 : Inport  Port=2
  In3 : Inport  Port=3
  In4 : Inport  Port=4
  In5 : Inport  Port=5
  In6 : Inport  Port=6
  Demux : Demux  Outputs=2
  Demux1 : Demux  Outputs=2
  Demux2 : Demux  Outputs=2
  Mux : Mux  Inputs=9
  Vector Concatenate : Concatenate
  Vector Concatenate1 : Concatenate
  Vector Concatenate2 : Concatenate
  Out4 : Outport
  Out1 : Outport  Port=2
  Out2 : Outport  Port=3
  Out3 : Outport  Port=4
  wires:
  In3/1 -> Mux/9, Vector Concatenate2/2
  In1/1 -> Mux/3, Vector Concatenate/2
  In4/1 -> Demux/1, Vector Concatenate/1
  Vector Concatenate2/1 -> Out3/1
  Vector Concatenate1/1 -> Out2/1
  Vector Concatenate/1 -> Out1/1
  In5/1 -> Demux1/1, Vector Concatenate1/1
  In2/1 -> Mux/6, Vector Concatenate1/2
  In6/1 -> Demux2/1, Vector Concatenate2/1
  Mux/1 -> Out4/1
  Demux/1 -> Mux/1
  Demux/2 -> Mux/2
  Demux1/1 -> Mux/4
  Demux1/2 -> Mux/5
  Demux2/1 -> Mux/7
  Demux2/2 -> Mux/8

== system LoFT_Example3/FOWT System/Subsystem5/FOWT8/wind speed(m//s) ==
  Inflow : Inport
  In2 : Inport  Port=2
  Add : Sum
  Demux : Demux  Outputs=3
  Product : Product
  Trigonometric Function : Trigonometry  Operator=cos
  add : Sum  Inputs=+-
  add1 : Sum  Inputs=+-
  hub height : Gain  Gain=145
  smooth1 : Subsystem  Commented=on
  Effective : Outport
  Measured : Outport  Port=2
  FB : Outport  Port=3
  wires:
  Inflow/1 -> add/1, add1/1
  [HubVelocity] -> FB/1
  [HubVelocity] -> add/2
  [HubVelocity] -> add1/2
  Add/1 -> [HubVelocity]
  Product/1 -> Add/2
  add1/1 -> Measured/1
  add/1 -> Effective/1
  Demux/3 -> Trigonometric Function/1, hub height/1
  Demux/1 -> Add/1
  Trigonometric Function/1 -> Product/2
  hub height/1 -> Product/1
  In2/1 -> Demux/1

== system LoFT_Example3/FOWT System/Subsystem5/FOWT9/Aerodynamics and Local Control Systems ==
  WindSpeed : Inport
  "Measureed " : Inport  Port=2
  Nacelle Speed : Inport  Port=3
  Power : Inport  Port=4
  Blade Pitch : Inport  Port=5
  Switch : Inport  Port=6
  Constant1 : Constant  Value=90*pi/180
  Demux : Demux  Outputs=2
  Divide3 : Product  Inputs=*/
  Hull Aerodynamic : Subsystem
  Local Control Systems : Subsystem
  Mux : Mux
  Mux1 : Mux
  Product : Product
  Rate Limiter : RateLimiter  RisingSlewLimit=Controller.torqueMaxRate  FallingSlewLimit=-Controller.torqueMaxRate  SampleTimeMode=inherited
  Rotor/drivetrain dynamics : Subsystem
  Saturation Dynamic : simulink/Discontinuities/Saturation Dynamic  OutMin=[]  OutMax=[]  OutDataTypeStr=Inherit: Same as second input  OutDataType=fixdt(1, 16)  OutScaling=2^-10  DoSatur=off
  Saturation2 : Saturate  UpperLimit=Controller.torqueMax  LowerLimit=0
  Switch1 : Switch  Criteria=u2 > Threshold  SaturateOnIntegerOverflow=off  InputSameDT=off
  Transfer Fcn : TransferFcn  Denominator=[0.2 1]
  smooth1 : Subsystem
  wind speed estimator : Subsystem
  Nacelle : Outport
  drivetrain : Outport  Port=2
  F_aero : Outport  Port=3
  wires:
  Transfer Fcn/1 -> [BldPitch]
  Mux1/1 -> drivetrain/1
  Mux/1 -> Nacelle/1
  Local Control Systems/2(BldPitch) -> Saturation Dynamic/2
  Saturation Dynamic/1 -> Transfer Fcn/1
  Switch/1 -> Demux/1
  [RotSpeed] -> Divide3/2
  Rate Limiter/1 -> Saturation2/1
  Switch1/1 -> Rate Limiter/1
  Local Control Systems/1(GenTorq) -> Switch1/3
  Divide3/1 -> Switch1/1
  Nacelle Speed/1 -> Local Control Systems/3(Nacelle Speed)
  [RotSpeed] -> Local Control Systems/2(RotSpeed)
  Power/1 -> smooth1/1(In1)
  Blade Pitch/1 -> Saturation Dynamic/3
  Saturation2/1 -> [GenTorq]
  smooth1/1(Out1) -> Divide3/1
  WindSpeed/1 -> [EffectiveWS]
  [EffectiveWS] -> Hull Aerodynamic/1(In1)
  [RotSpeed] -> Hull Aerodynamic/2(In2)
  [BldPitch] -> Hull Aerodynamic/3(In4)
  Hull Aerodynamic/1(Out1) -> F_aero/1
  [RotSpeed] -> Rotor/drivetrain dynamics/1(In1)
  [EffectiveWS] -> Rotor/drivetrain dynamics/2(In2)
  [BldPitch] -> Rotor/drivetrain dynamics/3(In3)
  [EffectiveWS] -> Rotor/drivetrain dynamics/4(In4)
  [GenTorq] -> Rotor/drivetrain dynamics/5(In5)
  Rotor/drivetrain dynamics/1(Out1) -> [RotSpeed]
  [EffectiveWS] -> Mux/1
  [MeasuredWS] -> Local Control Systems/1(WindSpeed)
  "Measureed "/1 -> [MeasuredWS]
  [MeasuredWS] -> wind speed estimator/1(In1)
  wind speed estimator/1(Out1) -> Mux/2
  [BldPitch] -> Mux/4
  Hull Aerodynamic/2(Rotor thrust) -> [RotorThrust]
  [RotorThrust] -> Mux/3
  Demux/1 -> Switch1/2
  [RotSpeed] -> Mux1/1, Product/1
  [GenTorq] -> Mux1/2, Product/2
  Product/1 -> Mux1/3
  Rotor/drivetrain dynamics/2(Out2) -> [RotTorq]
  [RotTorq] -> Mux1/4
  Constant1/1 -> Saturation Dynamic/1

== system LoFT_Example3/FOWT System/Subsystem5/FOWT9/Hydrodynamics ==
  Acceleration : Inport
  Speed : Inport  Port=2
  Position : Inport  Port=3
  Wave : Inport  Port=4
  Add : Sum  Inputs=--+
  excitation force : Subsystem
  radiation force : Subsystem
  "viscous force " : Subsystem
  Out1 : Outport
  wires:
  Wave/1 -> excitation force/2(Wave)
  Add/1 -> Out1/1
  excitation force/1(Fext) -> Add/3
  "viscous force "/1(F_vis) -> Add/2
  radiation force/1(F_rad) -> Add/1
  Position/1 -> excitation force/1(position)
  Acceleration/1 -> radiation force/1(velocity)
  Speed/1 -> "viscous force "/1(In1), radiation force/2(In2)

== system LoFT_Example3/FOWT System/Subsystem5/FOWT9/Hydrostatics ==
  position : Inport
  Add : Sum
  Add2 : Sum  Inputs=+--
  Assignment : Assignment  DiagnosticForDimensions=Warning  IndexOptions=Index vector (dialog)  Indices=2  OutputSizes=1
  Constant : Constant  Value=Property.masstot-9.7e6
  Constant1 : Constant  Value=Property.volume
  Constant2 : Constant  Value=[0 0 0]
  Constant3 : Constant  Value=4*445087
  Product : Product  Multiplication=Matrix(*)
  "Surge,heave,pitch, Hydro stiffness (3×3)" : Constant  Value=Hydro.hydrostatic
  rho * g : Gain  Gain=1025*9.81
  rho * g1 : Gain  Gain=9.81
  Out1 : Outport
  wires:
  Add2/1 -> Assignment/2
  Add/1 -> Out1/1
  Assignment/1 -> Add/1
  Constant2/1 -> Assignment/1
  rho * g/1 -> Add2/2
  rho * g1/1 -> Add2/1
  Constant/1 -> rho * g1/1
  Product/1 -> Add/2
  Constant1/1 -> rho * g/1
  position/1 -> Product/2
  "Surge,heave,pitch, Hydro stiffness (3×3)"/1 -> Product/1
  Constant3/1 -> Add2/3

== system LoFT_Example3/FOWT System/Subsystem5/FOWT9/Measurements ==
  Nacelle : Inport
  drivetrain : Inport  Port=2
  platform : Inport  Port=3
  Bus Creator : BusCreator  Inputs=17
  Demux : Demux  Outputs=9
  Demux1 : Demux
  Demux2 : Demux
  Out1 : Outport
  wires:
  drivetrain/1 -> Demux2/1
  Demux2/4 -> Bus Creator/8  "RotTorq"
  Demux2/3 -> Bus Creator/7  "GenPwr"
  Demux2/2 -> Bus Creator/6  "GenTorq"
  Demux2/1 -> Bus Creator/5  "RotSpeed"
  Demux/1 -> Bus Creator/9  "PtfmSurge"
  Demux/2 -> Bus Creator/10  "PtfmHeave"
  Demux/3 -> Bus Creator/11  "PtfmPitch"
  Demux/4 -> Bus Creator/12  "PtfmTVxi"
  Demux/5 -> Bus Creator/13  "PtfmTVzi"
  Demux/6 -> Bus Creator/14  "PtfmRVyi"
  Demux/7 -> Bus Creator/15  "PtfmTAxi"
  Demux/8 -> Bus Creator/16  "PtfmTAzi"
  Demux/9 -> Bus Creator/17  "PtfmRAyi"
  Demux1/1 -> Bus Creator/1  "WindVelX"
  Demux1/2 -> Bus Creator/2  "WindEst"
  Demux1/3 -> Bus Creator/3  "RotThrust"
  Demux1/4 -> Bus Creator/4  "BldPitch"
  Bus Creator/1 -> Out1/1
  Nacelle/1 -> Demux1/1
  platform/1 -> Demux/1

== system LoFT_Example3/FOWT System/Subsystem5/FOWT9/Moorings ==
  position : Inport
  2-D Lookup Table : Lookup_n-D  NumberOfTableDimensions=3  BreakpointsForDimension1=Mooring.X  BreakpointsForDimension2=Mooring.Z  BreakpointsForDimension3=Mooring.RY  Table=Mooring.FX  InternalRulePriority=Speed  RndMeth=Simplest
      settings: InputPortMap=u0,u1,u2
  2-D Lookup Table3 : Lookup_n-D  NumberOfTableDimensions=3  BreakpointsForDimension1=LoFT.Mooring.X  BreakpointsForDimension2=LoFT.Mooring.Z  BreakpointsForDimension3=LoFT.Mooring.RY  Table=LoFT.Mooring.FZ  InternalRulePriority=Speed  RndMeth=Simplest
      settings: InputPortMap=u0,u1,u2
  2-D Lookup Table4 : Lookup_n-D  NumberOfTableDimensions=3  BreakpointsForDimension1=LoFT.Mooring.X  BreakpointsForDimension2=LoFT.Mooring.Z  BreakpointsForDimension3=LoFT.Mooring.RY  Table=LoFT.Mooring.MY  InternalRulePriority=Speed  RndMeth=Simplest
      settings: InputPortMap=u0,u1,u2
  Demux : Demux  Outputs=3
  Demux1 : Demux  Outputs=3
  Demux2 : Demux  Outputs=3
  Vector Concatenate1 : Concatenate  NumInputs=3
  Out1 : Outport
  wires:
  Vector Concatenate1/1 -> Out1/1
  Demux2/2 -> 2-D Lookup Table4/2
  Demux2/1 -> 2-D Lookup Table4/1
  2-D Lookup Table4/1 -> Vector Concatenate1/3
  2-D Lookup Table3/1 -> Vector Concatenate1/2
  Demux1/3 -> 2-D Lookup Table3/3
  Demux/2 -> 2-D Lookup Table/2
  Demux1/1 -> 2-D Lookup Table3/1
  Demux2/3 -> 2-D Lookup Table4/3
  Demux/1 -> 2-D Lookup Table/1
  position/1 -> Demux/1, Demux1/1, Demux2/1
  2-D Lookup Table/1 -> Vector Concatenate1/1
  Demux1/2 -> 2-D Lookup Table3/2
  Demux/3 -> 2-D Lookup Table/3

== system LoFT_Example3/FOWT System/Subsystem5/FOWT9/Subsystem1 ==
  In1 : Inport
  In2 : Inport  Port=2
  In3 : Inport  Port=3
  In4 : Inport  Port=4
  In5 : Inport  Port=5
  In6 : Inport  Port=6
  Demux : Demux  Outputs=2
  Demux1 : Demux  Outputs=2
  Demux2 : Demux  Outputs=2
  Mux : Mux  Inputs=9
  Vector Concatenate : Concatenate
  Vector Concatenate1 : Concatenate
  Vector Concatenate2 : Concatenate
  Out4 : Outport
  Out1 : Outport  Port=2
  Out2 : Outport  Port=3
  Out3 : Outport  Port=4
  wires:
  Demux2/2 -> Mux/8
  Demux2/1 -> Mux/7
  Demux1/2 -> Mux/5
  Demux1/1 -> Mux/4
  Demux/2 -> Mux/2
  Demux/1 -> Mux/1
  Mux/1 -> Out4/1
  In6/1 -> Vector Concatenate2/1, Demux2/1
  In2/1 -> Vector Concatenate1/2, Mux/6
  In5/1 -> Vector Concatenate1/1, Demux1/1
  Vector Concatenate/1 -> Out1/1
  Vector Concatenate1/1 -> Out2/1
  Vector Concatenate2/1 -> Out3/1
  In4/1 -> Vector Concatenate/1, Demux/1
  In1/1 -> Vector Concatenate/2, Mux/3
  In3/1 -> Vector Concatenate2/2, Mux/9

== system LoFT_Example3/FOWT System/Subsystem5/FOWT9/wind speed(m//s) ==
  Inflow : Inport
  In2 : Inport  Port=2
  Add : Sum
  Demux : Demux  Outputs=3
  Product : Product
  Trigonometric Function : Trigonometry  Operator=cos
  add : Sum  Inputs=+-
  add1 : Sum  Inputs=+-
  hub height : Gain  Gain=145
  smooth1 : Subsystem  Commented=on
  Effective : Outport
  Measured : Outport  Port=2
  FB : Outport  Port=3
  wires:
  In2/1 -> Demux/1
  hub height/1 -> Product/1
  Trigonometric Function/1 -> Product/2
  Demux/1 -> Add/1
  Demux/3 -> hub height/1, Trigonometric Function/1
  add/1 -> Effective/1
  add1/1 -> Measured/1
  Product/1 -> Add/2
  Add/1 -> [HubVelocity]
  [HubVelocity] -> add1/2
  [HubVelocity] -> add/2
  [HubVelocity] -> FB/1
  Inflow/1 -> add1/1, add/1

== system LoFT_Example3/FOWT System/Subsystem7/FOWT1/Aerodynamics and Local Control Systems ==
  WindSpeed : Inport
  "Measureed " : Inport  Port=2
  Nacelle Speed : Inport  Port=3
  Power : Inport  Port=4
  Blade Pitch : Inport  Port=5
  Switch : Inport  Port=6
  Constant1 : Constant  Value=90*pi/180
  Demux : Demux  Outputs=2
  Divide3 : Product  Inputs=*/
  Hull Aerodynamic : Subsystem
  Local Control Systems : Subsystem
  Mux : Mux
  Mux1 : Mux
  Product : Product
  Rate Limiter : RateLimiter  RisingSlewLimit=Controller.torqueMaxRate  FallingSlewLimit=-Controller.torqueMaxRate  SampleTimeMode=inherited
  Rotor/drivetrain dynamics : Subsystem
  Saturation Dynamic : simulink/Discontinuities/Saturation Dynamic  OutMin=[]  OutMax=[]  OutDataTypeStr=Inherit: Same as second input  OutDataType=fixdt(1, 16)  OutScaling=2^-10  DoSatur=off
  Saturation2 : Saturate  UpperLimit=Controller.torqueMax  LowerLimit=0
  Switch1 : Switch  Criteria=u2 > Threshold  SaturateOnIntegerOverflow=off  InputSameDT=off
  Transfer Fcn : TransferFcn  Denominator=[0.2 1]
  smooth1 : Subsystem
  wind speed estimator : Subsystem
  Nacelle : Outport
  drivetrain : Outport  Port=2
  F_aero : Outport  Port=3
  wires:
  Constant1/1 -> Saturation Dynamic/1
  [RotTorq] -> Mux1/4
  Rotor/drivetrain dynamics/2(Out2) -> [RotTorq]
  Product/1 -> Mux1/3
  [GenTorq] -> Product/2, Mux1/2
  [RotSpeed] -> Product/1, Mux1/1
  Demux/1 -> Switch1/2
  [RotorThrust] -> Mux/3
  Hull Aerodynamic/2(Rotor thrust) -> [RotorThrust]
  [BldPitch] -> Mux/4
  wind speed estimator/1(Out1) -> Mux/2
  [MeasuredWS] -> wind speed estimator/1(In1)
  "Measureed "/1 -> [MeasuredWS]
  [MeasuredWS] -> Local Control Systems/1(WindSpeed)
  [EffectiveWS] -> Mux/1
  Rotor/drivetrain dynamics/1(Out1) -> [RotSpeed]
  [GenTorq] -> Rotor/drivetrain dynamics/5(In5)
  [EffectiveWS] -> Rotor/drivetrain dynamics/4(In4)
  [BldPitch] -> Rotor/drivetrain dynamics/3(In3)
  [EffectiveWS] -> Rotor/drivetrain dynamics/2(In2)
  [RotSpeed] -> Rotor/drivetrain dynamics/1(In1)
  Hull Aerodynamic/1(Out1) -> F_aero/1
  [BldPitch] -> Hull Aerodynamic/3(In4)
  [RotSpeed] -> Hull Aerodynamic/2(In2)
  [EffectiveWS] -> Hull Aerodynamic/1(In1)
  WindSpeed/1 -> [EffectiveWS]
  smooth1/1(Out1) -> Divide3/1
  Saturation2/1 -> [GenTorq]
  Blade Pitch/1 -> Saturation Dynamic/3
  Power/1 -> smooth1/1(In1)
  [RotSpeed] -> Local Control Systems/2(RotSpeed)
  Nacelle Speed/1 -> Local Control Systems/3(Nacelle Speed)
  Divide3/1 -> Switch1/1
  Local Control Systems/1(GenTorq) -> Switch1/3
  Switch1/1 -> Rate Limiter/1
  Rate Limiter/1 -> Saturation2/1
  [RotSpeed] -> Divide3/2
  Switch/1 -> Demux/1
  Saturation Dynamic/1 -> Transfer Fcn/1
  Local Control Systems/2(BldPitch) -> Saturation Dynamic/2
  Mux/1 -> Nacelle/1
  Mux1/1 -> drivetrain/1
  Transfer Fcn/1 -> [BldPitch]

== system LoFT_Example3/FOWT System/Subsystem7/FOWT1/Hydrodynamics ==
  Acceleration : Inport
  Speed : Inport  Port=2
  Position : Inport  Port=3
  Wave : Inport  Port=4
  Add : Sum  Inputs=--+
  excitation force : Subsystem
  radiation force : Subsystem
  "viscous force " : Subsystem
  Out1 : Outport
  wires:
  Speed/1 -> radiation force/2(In2), "viscous force "/1(In1)
  Acceleration/1 -> radiation force/1(velocity)
  Position/1 -> excitation force/1(position)
  radiation force/1(F_rad) -> Add/1
  "viscous force "/1(F_vis) -> Add/2
  excitation force/1(Fext) -> Add/3
  Add/1 -> Out1/1
  Wave/1 -> excitation force/2(Wave)

== system LoFT_Example3/FOWT System/Subsystem7/FOWT1/Hydrostatics ==
  position : Inport
  Add : Sum
  Add2 : Sum  Inputs=+--
  Assignment : Assignment  DiagnosticForDimensions=Warning  IndexOptions=Index vector (dialog)  Indices=2  OutputSizes=1
  Constant : Constant  Value=Property.masstot-9.7e6
  Constant1 : Constant  Value=Property.volume
  Constant2 : Constant  Value=[0 0 0]
  Constant3 : Constant  Value=4*445087
  Product : Product  Multiplication=Matrix(*)
  "Surge,heave,pitch, Hydro stiffness (3×3)" : Constant  Value=Hydro.hydrostatic
  rho * g : Gain  Gain=1025*9.81
  rho * g1 : Gain  Gain=9.81
  Out1 : Outport
  wires:
  Constant3/1 -> Add2/3
  "Surge,heave,pitch, Hydro stiffness (3×3)"/1 -> Product/1
  position/1 -> Product/2
  Constant1/1 -> rho * g/1
  Product/1 -> Add/2
  Constant/1 -> rho * g1/1
  rho * g1/1 -> Add2/1
  rho * g/1 -> Add2/2
  Constant2/1 -> Assignment/1
  Assignment/1 -> Add/1
  Add/1 -> Out1/1
  Add2/1 -> Assignment/2
